simulink model "controller_sdfp_host"  (Simulink 7.3)
settings: Solver=ode45  StartTime=0.0  StopTime=2  RelTol=1e-3
values from neighbouring files (symbols this model uses):
  d = 16    [one_bit_control.m]
  fixpt_adder_in_bitwidth = w    (= 24)    [one_bit_control.m]
  fixpt_adder_in_position = d    (= 16)    [one_bit_control.m]
  fixpt_adder_out_bitwidth = w    (= 24)    [one_bit_control.m]
  fixpt_adder_out_position = d    (= 16)    [one_bit_control.m]
  fixpt_gain_bitwidth = w    (= 24)    [one_bit_control.m]
  fixpt_gain_position = d    (= 16)    [one_bit_control.m]
  k = 2^k_bitshift    (= 0.0001220703125)    [one_bit_control.m]
  p0 = (109.9*Ki)*T^3*k^-3    [one_bit_control.m]
  p1 = (20.78*Ki+109.9*Kp)*T^2*k^-2    [one_bit_control.m]
  p2 = (Ki+20.78*Kp)*T*k^-1    [one_bit_control.m]
  p3 = Kp    (= 8)    [one_bit_control.m]
  q0 = 0*T^3*k^-3    [one_bit_control.m]
  q1 = 174.8*T^2*k^-2    [one_bit_control.m]
  q2 = 26.33*T*k^-1    [one_bit_control.m]
  T = ts    [one_bit_control.m]
  ts = 1/Fs    [one_bit_control.m]
  ts_k_gain1 = k_bitshift - Fs_power_2    [one_bit_control.m]
  ts_k_gain2 = k_bitshift - Fs_power_2    [one_bit_control.m]
  ts_k_gain3 = k_bitshift - Fs_power_2    [one_bit_control.m]
  w = 24    [one_bit_control.m]
libraries: simulink x16, cstblocks x5, commnoisgen2 x1, simulink_extras x1
(part 1 of 2)
settings Model: Creator=Joseph Poverelli  LastModifiedBy=kunal
settings OptimizationCC: InitFltsAndDblsToZero=on

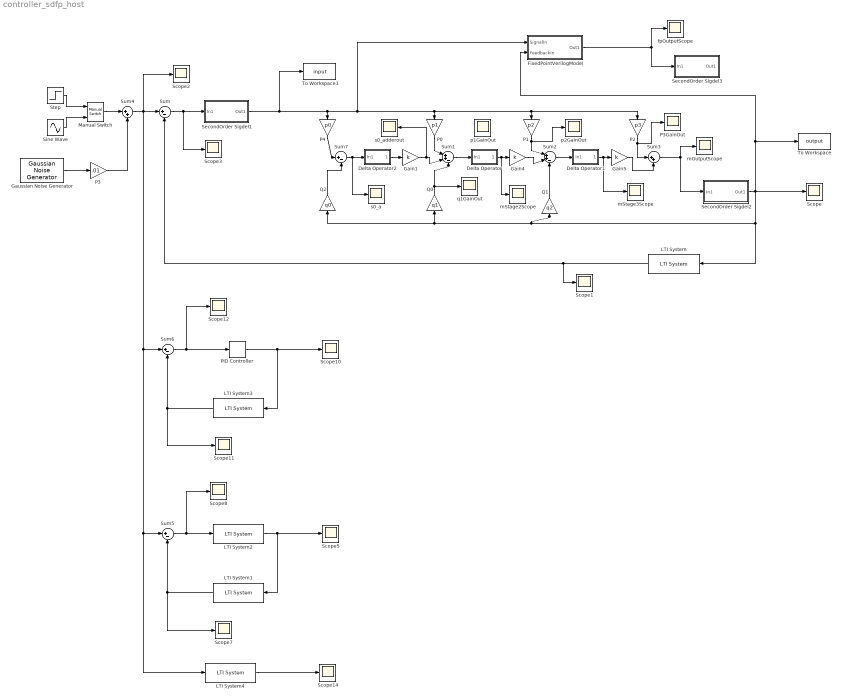
== system controller_sdfp_host ==
  Delta Operator : Subsystem
  Delta Operator1 : Subsystem
  Delta Operator2 : Subsystem
  FixedPointVerilogModel : Subsystem
  Gain1 : Gain  Gain=k  ParameterDataType=sfix(16)  ParameterScaling=2^0  OutDataType=fixdt(1,w,d)  RndMeth=Nearest
  Gain4 : Gain  Gain=k  ParameterDataType=sfix(16)  ParameterScaling=2^0  OutDataType=fixdt(1,w,d)  RndMeth=Nearest
  Gain5 : Gain  Gain=k  ParameterDataType=sfix(16)  ParameterScaling=2^0  OutDataType=fixdt(1,w,d)  RndMeth=Nearest
  Gaussian Noise Generator : commnoisgen2/Gaussian Noise Generator  SystemSampleTime=-1  m=0  d=1  s=41  Ts=T  frameBased=off  sampPerFrame=1  orient=off  outDataType=double
  LTI System{,1,3..4} (4 alike) : cstblocks/LTI System  SystemSampleTime=-1  sys=P  IC=[]
  LTI System2 : cstblocks/LTI System  SystemSampleTime=-1  sys=C  IC=[]
  Manual Switch : simulink/Signal Routing/Manual Switch  SystemSampleTime=-1  sw=0  action=0  varsize=off
  P0 : Gain  Gain=p1  ParameterDataType=sfix(16)  ParameterScaling=2^0  OutDataType=sfix(16)  OutScaling=2^0
  P1 : Gain  Gain=p2  ParameterDataType=sfix(16)  ParameterScaling=2^0  OutDataType=sfix(16)  OutScaling=2^0
  P2 : Gain  Gain=p3  ParameterDataType=sfix(16)  ParameterScaling=2^0  OutDataType=sfix(16)  OutScaling=2^0
  P3 : Gain  Gain=.01  ParameterDataType=sfix(16)  ParameterScaling=2^0  OutDataType=sfix(16)  OutScaling=2^0
  P3GainOut : Scope
      settings: YMin=-4  YMax=4  SaveName=ScopeData8
  P4 : Gain  Gain=p0  ParameterDataType=sfix(16)  ParameterScaling=2^0  OutDataType=sfix(16)  OutScaling=2^0
  PID Controller : simulink_extras/Additional Linear/PID Controller  SystemSampleTime=-1  P=10  I=100  D=.1
  Q0 : Gain  Gain=q1  ParameterDataType=sfix(16)  ParameterScaling=2^0  OutDataType=sfix(16)  OutScaling=2^0
  Q1 : Gain  Gain=q2  ParameterDataType=sfix(16)  ParameterScaling=2^0  OutDataType=sfix(16)  OutScaling=2^0
  Q2 : Gain  Gain=q0  ParameterDataType=sfix(16)  ParameterScaling=2^0  OutDataType=sfix(16)  OutScaling=2^0
  Scope{,1..3,5,7..8,10..12,14} (11 alike) : Scope
      Scope settings: YMin=-1  YMax=1  SaveName=Y  DataFormat=Structure  SampleInput=on  SampleTime=ts
      Scope1 settings: YMin=-0.10575  YMax=-0.1035  SaveName=plant_output  DataFormat=Structure  SampleInput=on  SampleTime=ts
      Scope10 settings: YMin=-10  YMax=10  SaveName=Y1  DataFormat=Structure  SampleInput=on  SampleTime=ts
      Scope11 settings: YMin=0.01  YMax=0.0325  SaveName=continuous_plant_output1  DataFormat=Structure  SampleInput=on  SampleTime=ts
      Scope12 settings: YMin=-10  YMax=10  SaveName=Y2  DataFormat=Array  SampleInput=on  SampleTime=ts
      Scope14 settings: YMin=1.075  YMax=1.45  SaveName=Y4  DataFormat=Structure  SampleInput=on  SampleTime=ts
      Scope2 settings: YMin=0.06375  YMax=0.06575  SaveName=in  DataFormat=Structure  SampleInput=on  SampleTime=ts
      Scope3 settings: YMin=0.06375  YMax=0.06575  SaveName=error  DataFormat=Array  SampleInput=on  SampleTime=ts
      Scope5 settings: YMin=-10  YMax=10  SaveName=Y3  DataFormat=Structure  SampleInput=on  SampleTime=ts
      Scope7 settings: YMin=0.2795  YMax=0.283  SaveName=continuous_plant_output  DataFormat=Structure  SampleInput=on  SampleTime=ts
      Scope8 settings: YMin=-10  YMax=10  SaveName=Y6  DataFormat=Array  SampleInput=on  SampleTime=ts
  SecondOrder Sigdel1 : Subsystem
  SecondOrder Sigdel2 : Subsystem
  SecondOrder Sigdel3 : Subsystem
  Sine Wave : Sin  Amplitude=.25  Bias=0  Frequency=2*pi*1  Phase=0  Samples=10  SampleTime=0  Offset=0
  Step : Step  After=.1  SampleTime=ts
  Sum : Sum  Inputs=|+-  OutDataType=sfix(16)  OutScaling=2^0
  Sum1 : Sum  Inputs=|++-  OutDataType=fixdt(1,w,d)  RndMeth=Nearest
  Sum2 : Sum  Inputs=|++-  OutDataType=fixdt(1,w,d)  RndMeth=Nearest
  Sum3 : Sum  Inputs=|++  OutMin=[-p2]  OutMax=[p2]  OutDataType=fixdt(1,w,d)  RndMeth=Nearest  SaturateOnIntegerOverflow=on
  Sum4 : Sum  Inputs=|++  OutDataType=sfix(16)  OutScaling=2^0
  Sum5 : Sum  Inputs=|+-  OutDataType=sfix(16)  OutScaling=2^0
  Sum6 : Sum  Inputs=|+-  OutDataType=sfix(16)  OutScaling=2^0
  Sum7 : Sum  Inputs=|+-  OutDataType=fixdt(1,w,d)  RndMeth=Nearest
  To Workspace : ToWorkspace  VariableName=output  SampleTime=-1  SaveFormat=Array
  To Workspace1 : ToWorkspace  VariableName=input  SampleTime=-1  SaveFormat=Array
  fpOutputScope : Scope
      settings: YMin=-9.97  YMax=-9.8  SaveName=c_output1  DataFormat=Structure  SampleInput=on  SampleTime=ts
  mOutputScope : Scope
      settings: YMin=-9.97  YMax=-9.8  SaveName=c_output  DataFormat=Structure  SampleInput=on  SampleTime=ts
  mStage2Scope : Scope
      settings: YMin=-0.175  YMax=0.025  SaveName=delta3  DataFormat=Array  SampleInput=on  SampleTime=ts
  mStage3Scope : Scope
      settings: YMin=-0.225  YMax=0.025  SaveName=delta  DataFormat=Array  SampleInput=on  SampleTime=ts
  p1GainOut : Scope
      settings: YMin=-4  YMax=4  SaveName=ScopeData5
  p2GainOut : Scope
      settings: YMin=-4  YMax=4  SaveName=ScopeData7
  q1GainOut : Scope
      settings: YMin=-0.75  YMax=0.75  SaveName=ScopeData13
  s0_a : Scope
      settings: YMin=-0.1  YMax=0.1  SaveName=ScopeData4
  s0_adderout : Scope
      settings: YMin=-5e-08  YMax=5e-07  SaveName=ScopeData12
  wires:
  Sum/1 -> SecondOrder Sigdel1/1(In1), Scope3/1
  LTI System/1 -> Sum/2, Scope1/1
  SecondOrder Sigdel1/1(Out1) -> P4/1, P0/1, P1/1, P2/1, FixedPointVerilogModel/1(SignalIn), To Workspace1/1
  Sum3/1 -> mOutputScope/1, SecondOrder Sigdel2/1(In1)
  P0/1 -> Sum1/1
  Q1/1 -> Sum2/3
  P1/1 -> Sum2/1, p2GainOut/1
  P2/1 -> Sum3/1, P3GainOut/1
  Gain5/1 -> Sum3/2
  SecondOrder Sigdel2/1(Out1) -> LTI System/1, Q1/1, Q0/1, Q2/1, Scope/1, To Workspace/1, FixedPointVerilogModel/2(FeedbackIn)
  Delta Operator/1(Out1) -> mStage2Scope/1, Gain4/1
  Sum1/1 -> Delta Operator/1(In1)
  Sum2/1 -> Delta Operator1/1(In1)
  Delta Operator1/1(Out1) -> Gain5/1, mStage3Scope/1
  Manual Switch/1 -> Sum4/1
  Gaussian Noise Generator/1 -> P3/1
  Sum4/1 -> Sum/1, Scope2/1, Sum6/1, Sum5/1, LTI System4/1
  P3/1 -> Sum4/2
  Sum5/1 -> Scope8/1, LTI System2/1
  LTI System1/1 -> Sum5/2, Scope7/1
  Sine Wave/1 -> Manual Switch/2
  Step/1 -> Manual Switch/1
  LTI System2/1 -> LTI System1/1, Scope5/1
  Sum6/1 -> Scope12/1, PID Controller/1
  LTI System3/1 -> Sum6/2, Scope11/1
  PID Controller/1 -> LTI System3/1, Scope10/1
  P4/1 -> Sum7/1
  Q2/1 -> Sum7/2
  Delta Operator2/1(Out1) -> Gain1/1
  Sum7/1 -> Delta Operator2/1(In1), s0_a/1
  Q0/1 -> Sum1/3, q1GainOut/1
  Gain1/1 -> Sum1/2, s0_adderout/1
  Gain4/1 -> Sum2/2
  LTI System4/1 -> Scope14/1
  FixedPointVerilogModel/1(Out1) -> fpOutputScope/1, SecondOrder Sigdel3/1(In1)
  ? -> p1GainOut/1

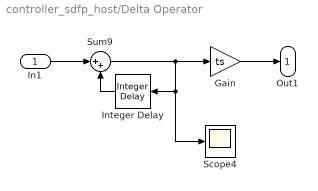
== system controller_sdfp_host/Delta Operator ==
  In1 : Inport  OutDataType=sfix(16)  OutScaling=2^0
  Gain : Gain  Gain=ts  ParameterDataType=sfix(16)  ParameterScaling=2^0  OutDataType=fixdt(1,w,d)  RndMeth=Nearest
  Integer Delay : simulink/Discrete/Integer Delay  vinit=0.0  samptime=-1  NumDelays=1
  Scope4 : Scope
      settings: YMin=-10  YMax=10  SaveName=delta1  DataFormat=Array  SampleInput=on  SampleTime=ts
  Sum9 : Sum  Inputs=|++  OutDataType=fixdt(1,w,d)  RndMeth=Nearest  SampleTime=ts
  Out1 : Outport  OutDataType=sfix(16)  OutScaling=2^0
  wires:
  In1/1 -> Sum9/1
  Sum9/1 -> Integer Delay/1, Scope4/1, Gain/1
  Integer Delay/1 -> Sum9/2
  Gain/1 -> Out1/1

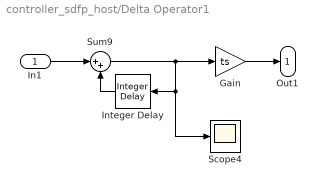
== system controller_sdfp_host/Delta Operator1 ==
  In1 : Inport  OutDataType=sfix(16)  OutScaling=2^0
  Gain : Gain  Gain=ts  ParameterDataType=sfix(16)  ParameterScaling=2^0  OutDataType=fixdt(1,w,d)  RndMeth=Nearest
  Integer Delay : simulink/Discrete/Integer Delay  vinit=0.0  samptime=-1  NumDelays=1
  Scope4 : Scope
      settings: YMin=-10  YMax=10  SaveName=delta2  DataFormat=Array  SampleInput=on  SampleTime=ts
  Sum9 : Sum  Inputs=|++  OutDataType=fixdt(1,w,d)  RndMeth=Nearest  SampleTime=ts
  Out1 : Outport  OutDataType=sfix(16)  OutScaling=2^0
  wires:
  In1/1 -> Sum9/1
  Sum9/1 -> Integer Delay/1, Scope4/1, Gain/1
  Integer Delay/1 -> Sum9/2
  Gain/1 -> Out1/1

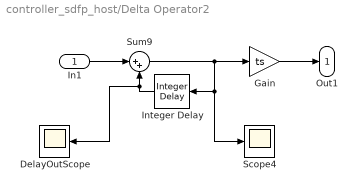
== system controller_sdfp_host/Delta Operator2 ==
  In1 : Inport  OutDataType=sfix(16)  OutScaling=2^0
  DelayOutScope : Scope
      settings: YMin=-900  YMax=700  SaveName=delta4  DataFormat=Array  SampleInput=on  SampleTime=ts
  Gain : Gain  Gain=ts  ParameterDataType=sfix(16)  ParameterScaling=2^0  OutDataType=fixdt(1,w,d)  RndMeth=Nearest
  Integer Delay : simulink/Discrete/Integer Delay  vinit=0.0  samptime=-1  NumDelays=1
  Scope4 : Scope
      settings: YMin=-100  YMax=1000  SaveName=delta43  DataFormat=Array  SampleInput=on  SampleTime=ts
  Sum9 : Sum  Inputs=|++  OutDataType=fixdt(1,w,d)  RndMeth=Nearest  SampleTime=ts
  Out1 : Outport  OutDataType=sfix(16)  OutScaling=2^0
  wires:
  In1/1 -> Sum9/1
  Sum9/1 -> Integer Delay/1, Scope4/1, Gain/1
  Integer Delay/1 -> Sum9/2, DelayOutScope/1
  Gain/1 -> Out1/1

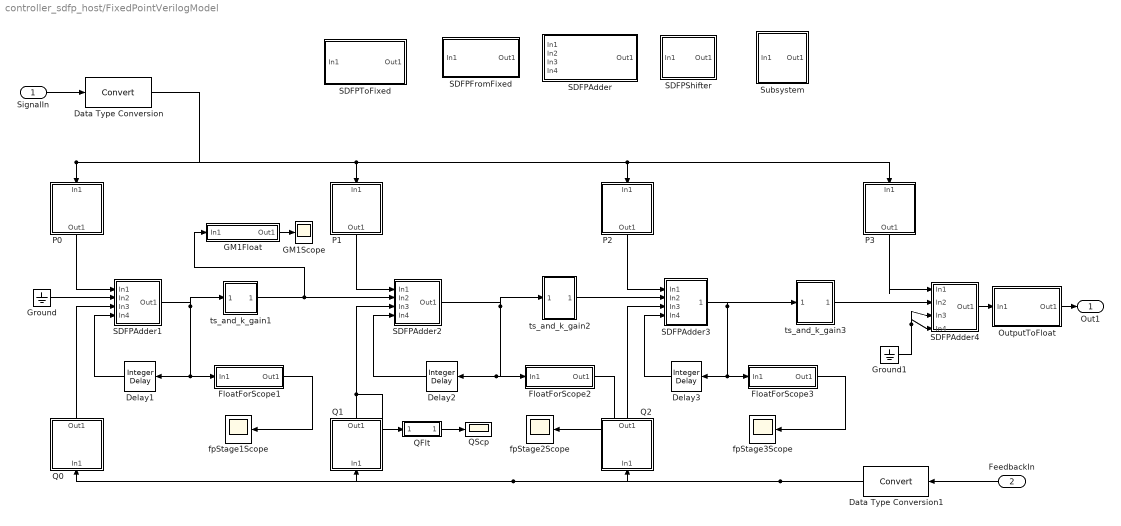
== system controller_sdfp_host/FixedPointVerilogModel ==
  SignalIn : Inport  OutDataType=fixdt(1, 16)  OutScaling=2^0
  FeedbackIn : Inport  Port=2  OutDataType=fixdt(1, 16)  OutScaling=2^0
  Data Type Conversion : DataTypeConversion  OutDataType=fixdt(1, 16)  OutScaling=2^0
  Data Type Conversion1 : DataTypeConversion  OutDataType=fixdt(1, 16)  OutScaling=2^0
  Delay1 : simulink/Discrete/Integer Delay  vinit=0.0  samptime=-1  NumDelays=1
  Delay2 : simulink/Discrete/Integer Delay  vinit=0.0  samptime=-1  NumDelays=1
  Delay3 : simulink/Discrete/Integer Delay  vinit=0.0  samptime=-1  NumDelays=1
  FloatForScope1 : Subsystem  mask{bitwidth=fixpt_adder_out_bitwidth, fp_position=fixpt_adder_out_position}
      mask prompts: bitwidth "Input Bitwidth"; fp_position "Input Point Position"
      mask Display: disp('Fixed -> Float');
  FloatForScope2 : Subsystem  mask{bitwidth=fixpt_adder_out_bitwidth, fp_position=fixpt_adder_out_position}
      mask prompts: bitwidth "Input Bitwidth"; fp_position "Input Point Position"
      mask Display: disp('Fixed -> Float');
  FloatForScope3 : Subsystem  mask{bitwidth=fixpt_adder_out_bitwidth, fp_position=fixpt_adder_out_position}
      mask prompts: bitwidth "Input Bitwidth"; fp_position "Input Point Position"
      mask Display: disp('Fixed -> Float');
  GM1Float : Subsystem  mask{bitwidth=fixpt_gain_bitwidth, fp_position=fixpt_gain_position}
      mask prompts: bitwidth "Input Bitwidth"; fp_position "Input Point Position"
      mask Display: disp('Fixed -> Float');
  GM1Scope : Scope
      settings: YMin=-1.75e-05  YMax=0  SaveName=ScopeData6
  Ground : Ground
  Ground1 : Ground
  OutputToFloat : Subsystem  mask{bitwidth=fixpt_adder_out_bitwidth, fp_position=fixpt_adder_out_position}
      mask prompts: bitwidth "Input Bitwidth"; fp_position "Input Point Position"
      mask Display: disp('Fixed -> Float');
  P0 : Subsystem  mask{gain=p0, bitwidth=fixpt_gain_bitwidth, fp_position=fixpt_gain_position}
      mask prompts: bitwidth "Output Bitwidth"; fp_position "Output Point Position"
      mask Display: plot([0.2 0.9 0.2 0.2],[0 .5 1 0]);disp('GainMux')
  P1 : Subsystem  mask{gain=p1, bitwidth=fixpt_gain_bitwidth, fp_position=fixpt_gain_position}
      mask prompts: bitwidth "Output Bitwidth"; fp_position "Output Point Position"
      mask Display: plot([0.2 0.9 0.2 0.2],[0 .5 1 0]);disp('GainMux')
  P2 : Subsystem  mask{gain=p2, bitwidth=fixpt_gain_bitwidth, fp_position=fixpt_gain_position}
      mask prompts: bitwidth "Output Bitwidth"; fp_position "Output Point Position"
      mask Display: plot([0.2 0.9 0.2 0.2],[0 .5 1 0]);disp('GainMux')
  P3 : Subsystem  mask{gain=p3, bitwidth=fixpt_gain_bitwidth, fp_position=fixpt_gain_position}
      mask prompts: bitwidth "Output Bitwidth"; fp_position "Output Point Position"
      mask Display: plot([0.2 0.9 0.2 0.2],[0 .5 1 0]);disp('GainMux')
  Q0 : Subsystem  mask{gain=q0, bitwidth=fixpt_gain_bitwidth, fp_position=fixpt_gain_position}
      mask prompts: bitwidth "Output Bitwidth"; fp_position "Output Point Position"
      mask Display: plot([0.2 0.9 0.2 0.2],[0 .5 1 0]);disp('GainMux')
  Q1 : Subsystem  mask{gain=q1, bitwidth=fixpt_gain_bitwidth, fp_position=fixpt_gain_position}
      mask prompts: bitwidth "Output Bitwidth"; fp_position "Output Point Position"
      mask Display: plot([0.2 0.9 0.2 0.2],[0 .5 1 0]);disp('GainMux')
  Q2 : Subsystem  mask{gain=q2, bitwidth=fixpt_gain_bitwidth, fp_position=fixpt_gain_position}
      mask prompts: bitwidth "Output Bitwidth"; fp_position "Output Point Position"
      mask Display: plot([0.2 0.9 0.2 0.2],[0 .5 1 0]);disp('GainMux')
  QFlt : Subsystem  mask{bitwidth=fixpt_gain_bitwidth, fp_position=fixpt_gain_position}
      mask prompts: bitwidth "Input Bitwidth"; fp_position "Input Point Position"
      mask Display: disp('Fixed -> Float');
  QScp : Scope
      settings: SaveName=ScopeData11
  SDFPAdder : Subsystem  mask{in_bitwidth=32, in_fp_position=8, out_bitwidth=32, out_fp_position=8}
      mask prompts: in_bitwidth "Input Bitwidth"; in_fp_position "Input Point Position"; out_bitwidth "Output Bitwidth"; out_fp_position "Output Point Position"
      mask Display: disp(['+\nSDFP'])
  SDFPAdder1 : Subsystem  mask{in_bitwidth=fixpt_adder_in_bitwidth, in_fp_position=fixpt_adder_in_position, out_bitwidth=fixpt_adder_out_bitwidth, out_fp_position=fixpt_adder_out_position}
      mask prompts: in_bitwidth "Input Bitwidth"; in_fp_position "Input Point Position"; out_bitwidth "Output Bitwidth"; out_fp_position "Output Point Position"
      mask Display: disp(['+\nSDFP'])
  SDFPAdder2 : Subsystem  mask{in_bitwidth=fixpt_adder_in_bitwidth, in_fp_position=fixpt_adder_in_position, out_bitwidth=fixpt_adder_out_bitwidth, out_fp_position=fixpt_adder_out_position}
      mask prompts: in_bitwidth "Input Bitwidth"; in_fp_position "Input Point Position"; out_bitwidth "Output Bitwidth"; out_fp_position "Output Point Position"
      mask Display: disp(['+\nSDFP'])
  SDFPAdder3 : Subsystem  mask{in_bitwidth=fixpt_adder_in_bitwidth, in_fp_position=fixpt_adder_in_position, out_bitwidth=fixpt_adder_out_bitwidth, out_fp_position=fixpt_adder_out_position}
      mask prompts: in_bitwidth "Input Bitwidth"; in_fp_position "Input Point Position"; out_bitwidth "Output Bitwidth"; out_fp_position "Output Point Position"
      mask Display: disp(['+\nSDFP'])
  SDFPAdder4 : Subsystem  mask{in_bitwidth=fixpt_adder_in_bitwidth, in_fp_position=fixpt_adder_in_position, out_bitwidth=fixpt_adder_out_bitwidth, out_fp_position=fixpt_adder_out_position}
      mask prompts: in_bitwidth "Input Bitwidth"; in_fp_position "Input Point Position"; out_bitwidth "Output Bitwidth"; out_fp_position "Output Point Position"
      mask Display: disp(['+\nSDFP'])
  SDFPFromFixed : Subsystem  mask{bitwidth=32, fp_position=16}
      mask prompts: bitwidth "Input Bitwidth"; fp_position "Input Point Position"
      mask Display: disp('Fixed -> Float');
  SDFPShifter : Subsystem  mask{shift_amount=1}
      mask init:
      | if(shift_amount > 0)
      |     dispval=sprintf('<< %d',shift_amount);
      | else
      |     dispval=sprintf('>> %d',-shift_amount);
      | end
      mask Display: disp(dispval);
  SDFPToFixed : Subsystem  mask{bitwidth=fixpt_adder_out_bitwidth, fp_position=fixpt_adder_out_position}
      mask prompts: bitwidth "Output Bitwidth"; fp_position "Output Point Position"
      mask Display: disp('Float -> Fixed')
  Subsystem : Subsystem  mask{gain=1.52, bitwidth=32, fp_position=16}
      mask prompts: bitwidth "Output Bitwidth"; fp_position "Output Point Position"
      mask Display: plot([0.2 0.9 0.2 0.2],[0 .5 1 0]);disp('GainMux')
  fpStage1Scope : Scope
      settings: YMin=-800  YMax=700
  fpStage2Scope : Scope
      settings: YMin=0  YMax=275
  fpStage3Scope : Scope
      settings: YMin=0  YMax=275  SaveName=ScopeData2
  ts_and_k_gain1 : Subsystem  mask{shift_amount=ts_k_gain1}
      mask init:
      | if(shift_amount > 0)
      |     dispval=sprintf('<< %d',shift_amount);
      | else
      |     dispval=sprintf('>> %d',-shift_amount);
      | end
      mask Display: disp(dispval);
  ts_and_k_gain2 : Subsystem  mask{shift_amount=ts_k_gain2}
      mask init:
      | if(shift_amount > 0)
      |     dispval=sprintf('<< %d',shift_amount);
      | else
      |     dispval=sprintf('>> %d',-shift_amount);
      | end
      mask Display: disp(dispval);
  ts_and_k_gain3 : Subsystem  mask{shift_amount=ts_k_gain3}
      mask init:
      | if(shift_amount > 0)
      |     dispval=sprintf('<< %d',shift_amount);
      | else
      |     dispval=sprintf('>> %d',-shift_amount);
      | end
      mask Display: disp(dispval);
  Out1 : Outport  OutDataType=fixdt(1, 16)  OutScaling=2^0
  wires:
  P0/1(Out1) -> SDFPAdder1/1(In1)
  Ground/1 -> SDFPAdder1/2(In2)
  Delay1/1 -> SDFPAdder1/4(In4)
  Q0/1(Out1) -> SDFPAdder1/3(In3)
  SDFPAdder1/1(Out1) -> Delay1/1, FloatForScope1/1(In1), ts_and_k_gain1/1(In1)
  P1/1(Out1) -> SDFPAdder2/1(In1)
  Delay2/1 -> SDFPAdder2/4(In4)
  Q1/1(Out1) -> SDFPAdder2/3(In3), QFlt/1(In1)
  SDFPAdder2/1(Out1) -> Delay2/1, FloatForScope2/1(In1), ts_and_k_gain2/1(In1)
  ts_and_k_gain1/1(Out1) -> SDFPAdder2/2(In2), GM1Float/1(In1)
  P2/1(Out1) -> SDFPAdder3/1(In1)
  Delay3/1 -> SDFPAdder3/4(In4)
  Q2/1(Out1) -> SDFPAdder3/3(In3)
  SDFPAdder3/1(Out1) -> ts_and_k_gain3/1(In1), Delay3/1, FloatForScope3/1(In1)
  ts_and_k_gain2/1(Out1) -> SDFPAdder3/2(In2)
  FeedbackIn/1 -> Data Type Conversion1/1
  Ground1/1 -> SDFPAdder4/4(In4), SDFPAdder4/3(In3)
  ts_and_k_gain3/1(Out1) -> SDFPAdder4/2(In2)
  P3/1(Out1) -> SDFPAdder4/1(In1)
  SDFPAdder4/1(Out1) -> OutputToFloat/1(In1)
  SignalIn/1 -> Data Type Conversion/1
  Data Type Conversion/1 -> P0/1(In1), P1/1(In1), P2/1(In1), P3/1(In1)
  Data Type Conversion1/1 -> Q2/1(In1), Q1/1(In1), Q0/1(In1)
  FloatForScope1/1(Out1) -> fpStage1Scope/1
  FloatForScope2/1(Out1) -> fpStage2Scope/1
  FloatForScope3/1(Out1) -> fpStage3Scope/1
  OutputToFloat/1(Out1) -> Out1/1
  QFlt/1(Out1) -> QScp/1
  GM1Float/1(Out1) -> GM1Scope/1

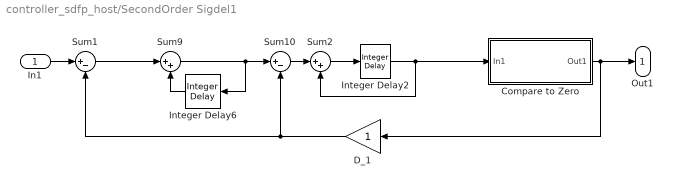
== system controller_sdfp_host/SecondOrder Sigdel1 ==
  In1 : Inport  OutDataType=sfix(16)  OutScaling=2^0
  Compare to Zero : Subsystem
  D_1 : Gain  ParameterDataType=sfix(16)  ParameterScaling=2^0  OutDataType=sfix(16)  OutScaling=2^0  SampleTime=ts
  Integer Delay2 : simulink/Discrete/Integer Delay  vinit=0.0  samptime=-1  NumDelays=1
  Integer Delay6 : simulink/Discrete/Integer Delay  vinit=0.0  samptime=-1  NumDelays=1
  Sum1 : Sum  Inputs=|+-  OutDataType=sfix(16)  OutScaling=2^0  SampleTime=ts
  Sum10 : Sum  Inputs=|+-  OutDataType=sfix(16)  OutScaling=2^0
  Sum2 : Sum  Inputs=|++  OutDataType=sfix(16)  OutScaling=2^0
  Sum9 : Sum  Inputs=|++  OutDataType=sfix(16)  OutScaling=2^0  SampleTime=ts
  Out1 : Outport  OutDataType=sfix(16)  OutScaling=2^0
  wires:
  Sum1/1 -> Sum9/1
  In1/1 -> Sum1/1
  Compare to Zero/1(Out1) -> D_1/1, Out1/1
  Sum2/1 -> Integer Delay2/1
  Integer Delay2/1 -> Sum2/2, Compare to Zero/1(In1)
  Sum9/1 -> Integer Delay6/1, Sum10/1
  Integer Delay6/1 -> Sum9/2
  Sum10/1 -> Sum2/1
  D_1/1 -> Sum1/2, Sum10/2

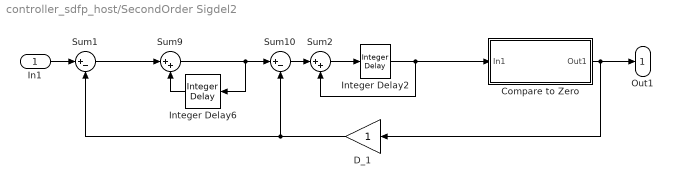
== system controller_sdfp_host/SecondOrder Sigdel2 ==
  In1 : Inport  OutDataType=sfix(16)  OutScaling=2^0
  Compare to Zero : Subsystem
  D_1 : Gain  ParameterDataType=sfix(16)  ParameterScaling=2^0  OutDataType=sfix(16)  OutScaling=2^0  SampleTime=ts
  Integer Delay2 : simulink/Discrete/Integer Delay  vinit=0.0  samptime=-1  NumDelays=1
  Integer Delay6 : simulink/Discrete/Integer Delay  vinit=0.0  samptime=-1  NumDelays=1
  Sum1 : Sum  Inputs=|+-  OutDataType=sfix(16)  OutScaling=2^0  SampleTime=ts
  Sum10 : Sum  Inputs=|+-  OutDataType=sfix(16)  OutScaling=2^0
  Sum2 : Sum  Inputs=|++  OutDataType=sfix(16)  OutScaling=2^0
  Sum9 : Sum  Inputs=|++  OutDataType=sfix(16)  OutScaling=2^0  SampleTime=ts
  Out1 : Outport  OutDataType=sfix(16)  OutScaling=2^0
  wires:
  Sum1/1 -> Sum9/1
  In1/1 -> Sum1/1
  Compare to Zero/1(Out1) -> D_1/1, Out1/1
  Sum2/1 -> Integer Delay2/1
  Integer Delay2/1 -> Sum2/2, Compare to Zero/1(In1)
  Sum9/1 -> Integer Delay6/1, Sum10/1
  Integer Delay6/1 -> Sum9/2
  Sum10/1 -> Sum2/1
  D_1/1 -> Sum1/2, Sum10/2

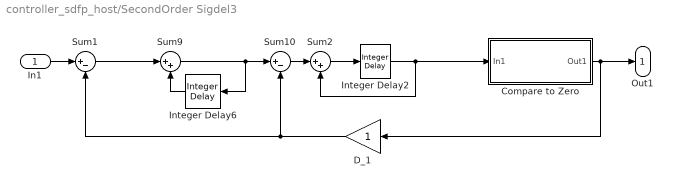
== system controller_sdfp_host/SecondOrder Sigdel3 ==
  In1 : Inport  OutDataType=sfix(16)  OutScaling=2^0
  Compare to Zero : Subsystem
  D_1 : Gain  ParameterDataType=sfix(16)  ParameterScaling=2^0  OutDataType=sfix(16)  OutScaling=2^0  SampleTime=ts
  Integer Delay2 : simulink/Discrete/Integer Delay  vinit=0.0  samptime=-1  NumDelays=1
  Integer Delay6 : simulink/Discrete/Integer Delay  vinit=0.0  samptime=-1  NumDelays=1
  Sum1 : Sum  Inputs=|+-  OutDataType=sfix(16)  OutScaling=2^0  SampleTime=ts
  Sum10 : Sum  Inputs=|+-  OutDataType=sfix(16)  OutScaling=2^0
  Sum2 : Sum  Inputs=|++  OutDataType=sfix(16)  OutScaling=2^0
  Sum9 : Sum  Inputs=|++  OutDataType=sfix(16)  OutScaling=2^0  SampleTime=ts
  Out1 : Outport  OutDataType=sfix(16)  OutScaling=2^0
  wires:
  Sum1/1 -> Sum9/1
  In1/1 -> Sum1/1
  Compare to Zero/1(Out1) -> D_1/1, Out1/1
  Sum2/1 -> Integer Delay2/1
  Integer Delay2/1 -> Sum2/2, Compare to Zero/1(In1)
  Sum9/1 -> Integer Delay6/1, Sum10/1
  Integer Delay6/1 -> Sum9/2
  Sum10/1 -> Sum2/1
  D_1/1 -> Sum1/2, Sum10/2

== system controller_sdfp_host/FixedPointVerilogModel/FloatForScope1 ==
  In1 : Inport  OutDataType=fixdt(1, 16)  OutScaling=2^0
  S-Function Builder : S-Function  InitFcn=try, set_param(gcb,'FunctionName','SDFPFromFixed'), end  FunctionName=SDFPFromFixed  Parameters=uint32(bitwidth),uint32(fp_position)  SFunctionModules=SDFPFromFixed_wrapper fpconv  WizardData=DataTag0  EnableBusSupport=off  mask(S-Function Builder){}
      mask help: The S-Function Builder block creates a wrapper C-MEX S-function from your supplied C code with multiple input ports, output ports, and a variable number of scalar, vector, or matrix parameters. The input and output ports can propagate Simulink built-in data types, fixed-point datatypes, complex, frame, 1-D, and 2-D signals. This block also supports discrete and continuous states of type real. You can optionally have the block generate a TLC file to be used with Real-Time Workshop for code generation.
      mask init:
      | val = [[.9  0.75 0.75 1 1 .9 .9 1]',[1 1 0.75 0.75 .9 .9 1 .9]'];try , sys = get_param(gcb,'SfunBuilderFcnName');if isempty(sys), sys = get_param(gcb,'FunctionName'); end,catch, sys = get_param(gcb,'FunctionName'); end
      settings: CopyFcn=set_param(gcbh,'LinkStatus','none')  PreSaveFcn=try, set_param(gcb,'FunctionName','SDFPFromFixed'), end  OpenFcn=sfunctionwizard(gcbh)
      mask Display: plot(val(:,1),val(:,2)),disp(sys)port_label('input',1,'fixed_in')port_label('output',1,'float_out')
  Out1 : Outport  OutDataType=fixdt(1, 16)  OutScaling=2^0
  wires:
  S-Function Builder/1 -> Out1/1
  In1/1 -> S-Function Builder/1

== system controller_sdfp_host/FixedPointVerilogModel/FloatForScope2 ==
  In1 : Inport  OutDataType=fixdt(1, 16)  OutScaling=2^0
  S-Function Builder : S-Function  InitFcn=try, set_param(gcb,'FunctionName','SDFPFromFixed'), end  FunctionName=SDFPFromFixed  Parameters=uint32(bitwidth),uint32(fp_position)  SFunctionModules=SDFPFromFixed_wrapper fpconv  WizardData=DataTag1  EnableBusSupport=off  mask(S-Function Builder){}
      mask help: The S-Function Builder block creates a wrapper C-MEX S-function from your supplied C code with multiple input ports, output ports, and a variable number of scalar, vector, or matrix parameters. The input and output ports can propagate Simulink built-in data types, fixed-point datatypes, complex, frame, 1-D, and 2-D signals. This block also supports discrete and continuous states of type real. You can optionally have the block generate a TLC file to be used with Real-Time Workshop for code generation.
      mask init: same as controller_sdfp_host/FixedPointVerilogModel/FloatForScope1/S-Function Builder
      settings: CopyFcn=set_param(gcbh,'LinkStatus','none')  PreSaveFcn=try, set_param(gcb,'FunctionName','SDFPFromFixed'), end  OpenFcn=sfunctionwizard(gcbh)
      mask Display: plot(val(:,1),val(:,2)),disp(sys)port_label('input',1,'fixed_in')port_label('output',1,'float_out')
  Out1 : Outport  OutDataType=fixdt(1, 16)  OutScaling=2^0
  wires:
  In1/1 -> S-Function Builder/1
  S-Function Builder/1 -> Out1/1

== system controller_sdfp_host/FixedPointVerilogModel/FloatForScope3 ==
  In1 : Inport  OutDataType=fixdt(1, 16)  OutScaling=2^0
  S-Function Builder : S-Function  InitFcn=try, set_param(gcb,'FunctionName','SDFPFromFixed'), end  FunctionName=SDFPFromFixed  Parameters=uint32(bitwidth),uint32(fp_position)  SFunctionModules=SDFPFromFixed_wrapper fpconv  WizardData=DataTag2  EnableBusSupport=off  mask(S-Function Builder){}
      mask help: The S-Function Builder block creates a wrapper C-MEX S-function from your supplied C code with multiple input ports, output ports, and a variable number of scalar, vector, or matrix parameters. The input and output ports can propagate Simulink built-in data types, fixed-point datatypes, complex, frame, 1-D, and 2-D signals. This block also supports discrete and continuous states of type real. You can optionally have the block generate a TLC file to be used with Real-Time Workshop for code generation.
      mask init: same as controller_sdfp_host/FixedPointVerilogModel/FloatForScope1/S-Function Builder
      settings: CopyFcn=set_param(gcbh,'LinkStatus','none')  PreSaveFcn=try, set_param(gcb,'FunctionName','SDFPFromFixed'), end  OpenFcn=sfunctionwizard(gcbh)
      mask Display: plot(val(:,1),val(:,2)),disp(sys)port_label('input',1,'fixed_in')port_label('output',1,'float_out')
  Out1 : Outport  OutDataType=fixdt(1, 16)  OutScaling=2^0
  wires:
  S-Function Builder/1 -> Out1/1
  In1/1 -> S-Function Builder/1

== system controller_sdfp_host/FixedPointVerilogModel/GM1Float ==
  In1 : Inport  OutDataType=fixdt(1, 16)  OutScaling=2^0
  S-Function Builder : S-Function  InitFcn=try, set_param(gcb,'FunctionName','SDFPFromFixed'), end  FunctionName=SDFPFromFixed  Parameters=uint32(bitwidth),uint32(fp_position)  SFunctionModules=SDFPFromFixed_wrapper fpconv  WizardData=DataTag3  EnableBusSupport=off  mask(S-Function Builder){}
      mask help: The S-Function Builder block creates a wrapper C-MEX S-function from your supplied C code with multiple input ports, output ports, and a variable number of scalar, vector, or matrix parameters. The input and output ports can propagate Simulink built-in data types, fixed-point datatypes, complex, frame, 1-D, and 2-D signals. This block also supports discrete and continuous states of type real. You can optionally have the block generate a TLC file to be used with Real-Time Workshop for code generation.
      mask init: same as controller_sdfp_host/FixedPointVerilogModel/FloatForScope1/S-Function Builder
      settings: CopyFcn=set_param(gcbh,'LinkStatus','none')  PreSaveFcn=try, set_param(gcb,'FunctionName','SDFPFromFixed'), end  OpenFcn=sfunctionwizard(gcbh)
      mask Display: plot(val(:,1),val(:,2)),disp(sys)port_label('input',1,'fixed_in')port_label('output',1,'float_out')
  Out1 : Outport  OutDataType=fixdt(1, 16)  OutScaling=2^0
  wires:
  In1/1 -> S-Function Builder/1
  S-Function Builder/1 -> Out1/1

== system controller_sdfp_host/FixedPointVerilogModel/OutputToFloat ==
  In1 : Inport  OutDataType=fixdt(1, 16)  OutScaling=2^0
  S-Function Builder : S-Function  InitFcn=try, set_param(gcb,'FunctionName','SDFPFromFixed'), end  FunctionName=SDFPFromFixed  Parameters=uint32(bitwidth),uint32(fp_position)  SFunctionModules=SDFPFromFixed_wrapper fpconv  WizardData=DataTag4  EnableBusSupport=off  mask(S-Function Builder){}
      mask help: The S-Function Builder block creates a wrapper C-MEX S-function from your supplied C code with multiple input ports, output ports, and a variable number of scalar, vector, or matrix parameters. The input and output ports can propagate Simulink built-in data types, fixed-point datatypes, complex, frame, 1-D, and 2-D signals. This block also supports discrete and continuous states of type real. You can optionally have the block generate a TLC file to be used with Real-Time Workshop for code generation.
      mask init: same as controller_sdfp_host/FixedPointVerilogModel/FloatForScope1/S-Function Builder
      settings: CopyFcn=set_param(gcbh,'LinkStatus','none')  PreSaveFcn=try, set_param(gcb,'FunctionName','SDFPFromFixed'), end  OpenFcn=sfunctionwizard(gcbh)
      mask Display: plot(val(:,1),val(:,2)),disp(sys)port_label('input',1,'fixed_in')port_label('output',1,'float_out')
  Out1 : Outport  OutDataType=fixdt(1, 16)  OutScaling=2^0
  wires:
  S-Function Builder/1 -> Out1/1
  In1/1 -> S-Function Builder/1

== system controller_sdfp_host/FixedPointVerilogModel/P0 ==
  In1 : Inport  OutDataType=fixdt(1, 16)  OutScaling=2^0
  S-Function Builder : S-Function  InitFcn=try, set_param(gcb,'FunctionName','SDFPGainSwitch'), end  FunctionName=SDFPGainSwitch  Parameters=single(gain),uint32(bitwidth),uint32(fp_position)  SFunctionModules=SDFPGainSwitch_wrapper fpconv  WizardData=DataTag5  EnableBusSupport=off  mask(S-Function Builder){}
      mask help: The S-Function Builder block creates a wrapper C-MEX S-function from your supplied C code with multiple input ports, output ports, and a variable number of scalar, vector, or matrix parameters. The input and output ports can propagate Simulink built-in data types, fixed-point datatypes, complex, frame, 1-D, and 2-D signals. This block also supports discrete and continuous states of type real. You can optionally have the block generate a TLC file to be used with Real-Time Workshop for code generation.
      mask init: same as controller_sdfp_host/FixedPointVerilogModel/FloatForScope1/S-Function Builder
      settings: CopyFcn=set_param(gcbh,'LinkStatus','none')  PreSaveFcn=try, set_param(gcb,'FunctionName','SDFPGainSwitch'), end  OpenFcn=sfunctionwizard(gcbh)
      mask Display: plot(val(:,1),val(:,2)),disp(sys)port_label('input',1,'sd_in')port_label('output',1,'gain_out')
  Out1 : Outport  OutDataType=fixdt(1, 16)  OutScaling=2^0
  wires:
  S-Function Builder/1 -> Out1/1
  In1/1 -> S-Function Builder/1

== system controller_sdfp_host/FixedPointVerilogModel/P1 ==
  In1 : Inport  OutDataType=fixdt(1, 16)  OutScaling=2^0
  Display : Display
      settings: Format=hex (Stored Integer)  Decimation=32
  Display1 : Display
      settings: Format=hex (Stored Integer)
  S-Function Builder : S-Function  InitFcn=try, set_param(gcb,'FunctionName','SDFPGainSwitch'), end  FunctionName=SDFPGainSwitch  Parameters=single(gain),uint32(bitwidth),uint32(fp_position)  SFunctionModules=SDFPGainSwitch_wrapper fpconv  WizardData=DataTag6  EnableBusSupport=off  mask(S-Function Builder){}
      mask help: The S-Function Builder block creates a wrapper C-MEX S-function from your supplied C code with multiple input ports, output ports, and a variable number of scalar, vector, or matrix parameters. The input and output ports can propagate Simulink built-in data types, fixed-point datatypes, complex, frame, 1-D, and 2-D signals. This block also supports discrete and continuous states of type real. You can optionally have the block generate a TLC file to be used with Real-Time Workshop for code generation.
      mask init: same as controller_sdfp_host/FixedPointVerilogModel/FloatForScope1/S-Function Builder
      settings: CopyFcn=set_param(gcbh,'LinkStatus','none')  PreSaveFcn=try, set_param(gcb,'FunctionName','SDFPGainSwitch'), end  OpenFcn=sfunctionwizard(gcbh)
      mask Display: plot(val(:,1),val(:,2)),disp(sys)port_label('input',1,'sd_in')port_label('output',1,'gain_out')port_label('output',2,'fixpt_out')port_label('output',3,'p_gain_out')
  Out1 : Outport  OutDataType=fixdt(1, 16)  OutScaling=2^0
  wires:
  In1/1 -> S-Function Builder/1
  S-Function Builder/1 -> Out1/1
  S-Function Builder/2 -> Display/1
  S-Function Builder/3 -> Display1/1

== system controller_sdfp_host/FixedPointVerilogModel/P2 ==
  In1 : Inport  OutDataType=fixdt(1, 16)  OutScaling=2^0
  S-Function Builder : S-Function  InitFcn=try, set_param(gcb,'FunctionName','SDFPGainSwitch'), end  FunctionName=SDFPGainSwitch  Parameters=single(gain),uint32(bitwidth),uint32(fp_position)  SFunctionModules=SDFPGainSwitch_wrapper fpconv  WizardData=DataTag7  EnableBusSupport=off  mask(S-Function Builder){}
      mask help: The S-Function Builder block creates a wrapper C-MEX S-function from your supplied C code with multiple input ports, output ports, and a variable number of scalar, vector, or matrix parameters. The input and output ports can propagate Simulink built-in data types, fixed-point datatypes, complex, frame, 1-D, and 2-D signals. This block also supports discrete and continuous states of type real. You can optionally have the block generate a TLC file to be used with Real-Time Workshop for code generation.
      mask init: same as controller_sdfp_host/FixedPointVerilogModel/FloatForScope1/S-Function Builder
      settings: CopyFcn=set_param(gcbh,'LinkStatus','none')  PreSaveFcn=try, set_param(gcb,'FunctionName','SDFPGainSwitch'), end  OpenFcn=sfunctionwizard(gcbh)
      mask Display: plot(val(:,1),val(:,2)),disp(sys)port_label('input',1,'sd_in')port_label('output',1,'gain_out')port_label('output',2,'fixpt_out')port_label('output',3,'p_gain_out')
  Out1 : Outport  OutDataType=fixdt(1, 16)  OutScaling=2^0
  wires:
  S-Function Builder/1 -> Out1/1
  In1/1 -> S-Function Builder/1

== system controller_sdfp_host/FixedPointVerilogModel/P3 ==
  In1 : Inport  OutDataType=fixdt(1, 16)  OutScaling=2^0
  S-Function Builder : S-Function  InitFcn=try, set_param(gcb,'FunctionName','SDFPGainSwitch'), end  FunctionName=SDFPGainSwitch  Parameters=single(gain),uint32(bitwidth),uint32(fp_position)  SFunctionModules=SDFPGainSwitch_wrapper fpconv  EnableBusSupport=off  mask(S-Function Builder){}
      mask help: The S-Function Builder block creates a wrapper C-MEX S-function from your supplied C code with multiple input ports, output ports, and a variable number of scalar, vector, or matrix parameters. The input and output ports can propagate Simulink built-in data types, fixed-point datatypes, complex, frame, 1-D, and 2-D signals. This block also supports discrete and continuous states of type real. You can optionally have the block generate a TLC file to be used with Real-Time Workshop for code generation.
      mask init: same as controller_sdfp_host/FixedPointVerilogModel/FloatForScope1/S-Function Builder
      settings: CopyFcn=set_param(gcbh,'LinkStatus','none')  PreSaveFcn=try, set_param(gcb,'FunctionName','SDFPGainSwitch'), end  OpenFcn=sfunctionwizard(gcbh)
      mask Display: plot(val(:,1),val(:,2)),disp(sys)port_label('input',1,'sd_in')port_label('output',1,'gain_out')
  Out1 : Outport  OutDataType=fixdt(1, 16)  OutScaling=2^0
  wires:
  S-Function Builder/1 -> Out1/1
  In1/1 -> S-Function Builder/1

== system controller_sdfp_host/FixedPointVerilogModel/Q0 ==
  In1 : Inport  OutDataType=fixdt(1, 16)  OutScaling=2^0
  S-Function Builder : S-Function  InitFcn=try, set_param(gcb,'FunctionName','SDFPGainSwitch'), end  FunctionName=SDFPGainSwitch  Parameters=single(gain),uint32(bitwidth),uint32(fp_position)  SFunctionModules=SDFPGainSwitch_wrapper fpconv  WizardData=DataTag8  EnableBusSupport=off  mask(S-Function Builder){}
      mask help: The S-Function Builder block creates a wrapper C-MEX S-function from your supplied C code with multiple input ports, output ports, and a variable number of scalar, vector, or matrix parameters. The input and output ports can propagate Simulink built-in data types, fixed-point datatypes, complex, frame, 1-D, and 2-D signals. This block also supports discrete and continuous states of type real. You can optionally have the block generate a TLC file to be used with Real-Time Workshop for code generation.
      mask init: same as controller_sdfp_host/FixedPointVerilogModel/FloatForScope1/S-Function Builder
      settings: CopyFcn=set_param(gcbh,'LinkStatus','none')  PreSaveFcn=try, set_param(gcb,'FunctionName','SDFPGainSwitch'), end  OpenFcn=sfunctionwizard(gcbh)
      mask Display: plot(val(:,1),val(:,2)),disp(sys)port_label('input',1,'sd_in')port_label('output',1,'gain_out')
  Out1 : Outport  OutDataType=fixdt(1, 16)  OutScaling=2^0
  wires:
  In1/1 -> S-Function Builder/1
  S-Function Builder/1 -> Out1/1

== system controller_sdfp_host/FixedPointVerilogModel/Q1 ==
  In1 : Inport  OutDataType=fixdt(1, 16)  OutScaling=2^0
  S-Function Builder : S-Function  InitFcn=try, set_param(gcb,'FunctionName','SDFPGainSwitch'), end  FunctionName=SDFPGainSwitch  Parameters=single(gain),uint32(bitwidth),uint32(fp_position)  SFunctionModules=SDFPGainSwitch_wrapper fpconv  EnableBusSupport=off  mask(S-Function Builder){}
      mask help: The S-Function Builder block creates a wrapper C-MEX S-function from your supplied C code with multiple input ports, output ports, and a variable number of scalar, vector, or matrix parameters. The input and output ports can propagate Simulink built-in data types, fixed-point datatypes, complex, frame, 1-D, and 2-D signals. This block also supports discrete and continuous states of type real. You can optionally have the block generate a TLC file to be used with Real-Time Workshop for code generation.
      mask init: same as controller_sdfp_host/FixedPointVerilogModel/FloatForScope1/S-Function Builder
      settings: CopyFcn=set_param(gcbh,'LinkStatus','none')  PreSaveFcn=try, set_param(gcb,'FunctionName','SDFPGainSwitch'), end  OpenFcn=sfunctionwizard(gcbh)
      mask Display: plot(val(:,1),val(:,2)),disp(sys)port_label('input',1,'sd_in')port_label('output',1,'gain_out')
  Out1 : Outport  OutDataType=fixdt(1, 16)  OutScaling=2^0
  wires:
  S-Function Builder/1 -> Out1/1
  In1/1 -> S-Function Builder/1

== system controller_sdfp_host/FixedPointVerilogModel/Q2 ==
  In1 : Inport  OutDataType=fixdt(1, 16)  OutScaling=2^0
  S-Function Builder : S-Function  InitFcn=try, set_param(gcb,'FunctionName','SDFPGainSwitch'), end  FunctionName=SDFPGainSwitch  Parameters=single(gain),uint32(bitwidth),uint32(fp_position)  SFunctionModules=SDFPGainSwitch_wrapper fpconv  WizardData=DataTag9  EnableBusSupport=off  mask(S-Function Builder){}
      mask help: The S-Function Builder block creates a wrapper C-MEX S-function from your supplied C code with multiple input ports, output ports, and a variable number of scalar, vector, or matrix parameters. The input and output ports can propagate Simulink built-in data types, fixed-point datatypes, complex, frame, 1-D, and 2-D signals. This block also supports discrete and continuous states of type real. You can optionally have the block generate a TLC file to be used with Real-Time Workshop for code generation.
      mask init: same as controller_sdfp_host/FixedPointVerilogModel/FloatForScope1/S-Function Builder
      settings: CopyFcn=set_param(gcbh,'LinkStatus','none')  PreSaveFcn=try, set_param(gcb,'FunctionName','SDFPGainSwitch'), end  OpenFcn=sfunctionwizard(gcbh)
      mask Display: plot(val(:,1),val(:,2)),disp(sys)port_label('input',1,'sd_in')port_label('output',1,'gain_out')
  Out1 : Outport  OutDataType=fixdt(1, 16)  OutScaling=2^0
  wires:
  In1/1 -> S-Function Builder/1
  S-Function Builder/1 -> Out1/1

== system controller_sdfp_host/FixedPointVerilogModel/QFlt ==
  In1 : Inport  OutDataType=fixdt(1, 16)  OutScaling=2^0
  S-Function Builder : S-Function  InitFcn=try, set_param(gcb,'FunctionName','SDFPFromFixed'), end  FunctionName=SDFPFromFixed  Parameters=uint32(bitwidth),uint32(fp_position)  SFunctionModules=SDFPFromFixed_wrapper fpconv  WizardData=DataTag10  EnableBusSupport=off  mask(S-Function Builder){}
      mask help: The S-Function Builder block creates a wrapper C-MEX S-function from your supplied C code with multiple input ports, output ports, and a variable number of scalar, vector, or matrix parameters. The input and output ports can propagate Simulink built-in data types, fixed-point datatypes, complex, frame, 1-D, and 2-D signals. This block also supports discrete and continuous states of type real. You can optionally have the block generate a TLC file to be used with Real-Time Workshop for code generation.
      mask init: same as controller_sdfp_host/FixedPointVerilogModel/FloatForScope1/S-Function Builder
      settings: CopyFcn=set_param(gcbh,'LinkStatus','none')  PreSaveFcn=try, set_param(gcb,'FunctionName','SDFPFromFixed'), end  OpenFcn=sfunctionwizard(gcbh)
      mask Display: plot(val(:,1),val(:,2)),disp(sys)port_label('input',1,'fixed_in')port_label('output',1,'float_out')
  Out1 : Outport  OutDataType=fixdt(1, 16)  OutScaling=2^0
  wires:
  In1/1 -> S-Function Builder/1
  S-Function Builder/1 -> Out1/1

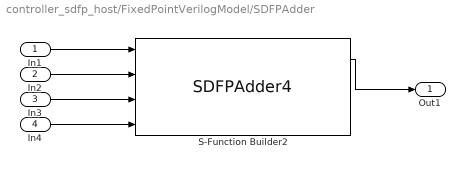
== system controller_sdfp_host/FixedPointVerilogModel/SDFPAdder ==
  In1 : Inport  OutDataType=fixdt(1, 16)  OutScaling=2^0
  In2 : Inport  Port=2  OutDataType=fixdt(1, 16)  OutScaling=2^0
  In3 : Inport  Port=3  OutDataType=fixdt(1, 16)  OutScaling=2^0
  In4 : Inport  Port=4  OutDataType=fixdt(1, 16)  OutScaling=2^0
  S-Function Builder2 : S-Function  InitFcn=try, set_param(gcb,'FunctionName','SDFPAdder4'), end  FunctionName=SDFPAdder4  Parameters=uint32(in_bitwidth),uint32(in_fp_position),uint32(out_bitwidth),uint32(out_fp_position)  SFunctionModules=SDFPAdder4_wrapper  WizardData=DataTag11  EnableBusSupport=off  mask(S-Function Builder){}
      mask help: The S-Function Builder block creates a wrapper C-MEX S-function from your supplied C code with multiple input ports, output ports, and a variable number of scalar, vector, or matrix parameters. The input and output ports can propagate Simulink built-in data types, fixed-point datatypes, complex, frame, 1-D, and 2-D signals. This block also supports discrete and continuous states of type real. You can optionally have the block generate a TLC file to be used with Real-Time Workshop for code generation.
      mask init: same as controller_sdfp_host/FixedPointVerilogModel/FloatForScope1/S-Function Builder
      settings: CopyFcn=set_param(gcbh,'LinkStatus','none')  PreSaveFcn=try, set_param(gcb,'FunctionName','SDFPAdder4'), end  OpenFcn=sfunctionwizard(gcbh)
      mask Display: plot(val(:,1),val(:,2)),disp(sys)port_label('input',1,'in0')port_label('input',2,'in1')port_label('input',3,'in2')port_label('input',4,'in3')port_label('output',1,'adder_out')
  Out1 : Outport  OutDataType=fixdt(1, 16)  OutScaling=2^0
  wires:
  In1/1 -> S-Function Builder2/1
  In2/1 -> S-Function Builder2/2
  In3/1 -> S-Function Builder2/3
  In4/1 -> S-Function Builder2/4
  S-Function Builder2/1 -> Out1/1

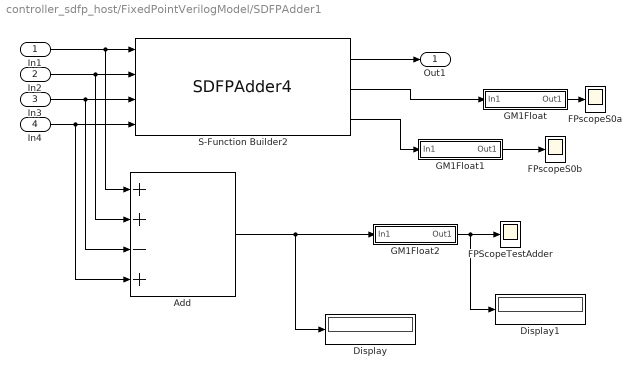
== system controller_sdfp_host/FixedPointVerilogModel/SDFPAdder1 ==
  In1 : Inport  OutDataType=fixdt(1, 16)  OutScaling=2^0
  In2 : Inport  Port=2  OutDataType=fixdt(1, 16)  OutScaling=2^0
  In3 : Inport  Port=3  OutDataType=fixdt(1, 16)  OutScaling=2^0
  In4 : Inport  Port=4  OutDataType=fixdt(1, 16)  OutScaling=2^0
  Add : Sum  Inputs=++-+  OutDataType=fixdt(1, 16)  OutScaling=2^-10
  Display : Display
      settings: Format=hex (Stored Integer)
  Display1 : Display
      settings: Decimation=5
  FPScopeTestAdder : Scope
      settings: YMin=-25  YMax=275  SaveName=ScopeData3
  FPscopeS0a : Scope
      settings: TimeRange=0.03999999999999998  YMin=-0.1  YMax=0.1  SaveName=ScopeData15
  FPscopeS0b : Scope
      settings: SaveName=ScopeData16
  GM1Float : Subsystem  mask{bitwidth=fixpt_gain_bitwidth, fp_position=fixpt_gain_position}
      mask prompts: bitwidth "Input Bitwidth"; fp_position "Input Point Position"
      mask Display: disp('Fixed -> Float');
  GM1Float1 : Subsystem  mask{bitwidth=fixpt_gain_bitwidth, fp_position=fixpt_gain_position}
      mask prompts: bitwidth "Input Bitwidth"; fp_position "Input Point Position"
      mask Display: disp('Fixed -> Float');
  GM1Float2 : Subsystem  mask{bitwidth=fixpt_adder_out_bitwidth, fp_position=fixpt_adder_out_position}
      mask prompts: bitwidth "Input Bitwidth"; fp_position "Input Point Position"
      mask Display: disp('Fixed -> Float');
  S-Function Builder2 : S-Function  InitFcn=try, set_param(gcb,'FunctionName','SDFPAdder4'), end  FunctionName=SDFPAdder4  Parameters=uint32(in_bitwidth),uint32(in_fp_position),uint32(out_bitwidth),uint32(out_fp_position)  SFunctionModules=SDFPAdder4_wrapper  WizardData=DataTag15  EnableBusSupport=off  mask(S-Function Builder){}
      mask help: The S-Function Builder block creates a wrapper C-MEX S-function from your supplied C code with multiple input ports, output ports, and a variable number of scalar, vector, or matrix parameters. The input and output ports can propagate Simulink built-in data types, fixed-point datatypes, complex, frame, 1-D, and 2-D signals. This block also supports discrete and continuous states of type real. You can optionally have the block generate a TLC file to be used with Real-Time Workshop for code generation.
      mask init: same as controller_sdfp_host/FixedPointVerilogModel/FloatForScope1/S-Function Builder
      settings: CopyFcn=set_param(gcbh,'LinkStatus','none')  PreSaveFcn=try, set_param(gcb,'FunctionName','SDFPAdder4'), end  OpenFcn=sfunctionwizard(gcbh)
      mask Display: plot(val(:,1),val(:,2)),disp(sys)port_label('input',1,'in0')port_label('input',2,'in1')port_label('input',3,'in2')port_label('input',4,'in3')port_label('output',1,'adder_out')port_label('output',2,'DBG_in01')port_label('output',3,'DBG_in012')
  Out1 : Outport  OutDataType=fixdt(1, 16)  OutScaling=2^0
  wires:
  In1/1 -> S-Function Builder2/1, Add/1
  In2/1 -> S-Function Builder2/2, Add/2
  In3/1 -> S-Function Builder2/3, Add/3
  In4/1 -> S-Function Builder2/4, Add/4
  S-Function Builder2/1 -> Out1/1
  GM1Float/1(Out1) -> FPscopeS0a/1
  S-Function Builder2/2 -> GM1Float/1(In1)
  GM1Float1/1(Out1) -> FPscopeS0b/1
  S-Function Builder2/3 -> GM1Float1/1(In1)
  Add/1 -> GM1Float2/1(In1), Display/1
  GM1Float2/1(Out1) -> FPScopeTestAdder/1, Display1/1

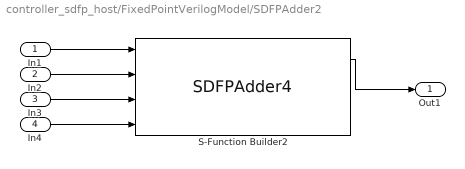
== system controller_sdfp_host/FixedPointVerilogModel/SDFPAdder2 ==
  In1 : Inport  OutDataType=fixdt(1, 16)  OutScaling=2^0
  In2 : Inport  Port=2  OutDataType=fixdt(1, 16)  OutScaling=2^0
  In3 : Inport  Port=3  OutDataType=fixdt(1, 16)  OutScaling=2^0
  In4 : Inport  Port=4  OutDataType=fixdt(1, 16)  OutScaling=2^0
  S-Function Builder2 : S-Function  InitFcn=try, set_param(gcb,'FunctionName','SDFPAdder4'), end  FunctionName=SDFPAdder4  Parameters=uint32(in_bitwidth),uint32(in_fp_position),uint32(out_bitwidth),uint32(out_fp_position)  SFunctionModules=SDFPAdder4_wrapper  WizardData=DataTag16  EnableBusSupport=off  mask(S-Function Builder){}
      mask help: The S-Function Builder block creates a wrapper C-MEX S-function from your supplied C code with multiple input ports, output ports, and a variable number of scalar, vector, or matrix parameters. The input and output ports can propagate Simulink built-in data types, fixed-point datatypes, complex, frame, 1-D, and 2-D signals. This block also supports discrete and continuous states of type real. You can optionally have the block generate a TLC file to be used with Real-Time Workshop for code generation.
      mask init: same as controller_sdfp_host/FixedPointVerilogModel/FloatForScope1/S-Function Builder
      settings: CopyFcn=set_param(gcbh,'LinkStatus','none')  PreSaveFcn=try, set_param(gcb,'FunctionName','SDFPAdder4'), end  OpenFcn=sfunctionwizard(gcbh)
      mask Display: plot(val(:,1),val(:,2)),disp(sys)port_label('input',1,'in0')port_label('input',2,'in1')port_label('input',3,'in2')port_label('input',4,'in3')port_label('output',1,'adder_out')
  Out1 : Outport  OutDataType=fixdt(1, 16)  OutScaling=2^0
  wires:
  S-Function Builder2/1 -> Out1/1
  In4/1 -> S-Function Builder2/4
  In3/1 -> S-Function Builder2/3
  In2/1 -> S-Function Builder2/2
  In1/1 -> S-Function Builder2/1
